simulink model "BMS_SOC_Estimation"  (R2026a)
settings: Solver=FixedStepDiscrete  StopTime=SIM_STOP_TIME  FixedStep=SIM_TIMESTEP
undefined symbols (not defined in the file): C1, DiscIntNeverNeededParam, OCV_values, Q_RATED, R0, R1, SIM_TIMESTEP, SOC_breakpoints, SOC_INIT
settings Model: VariantFading=off

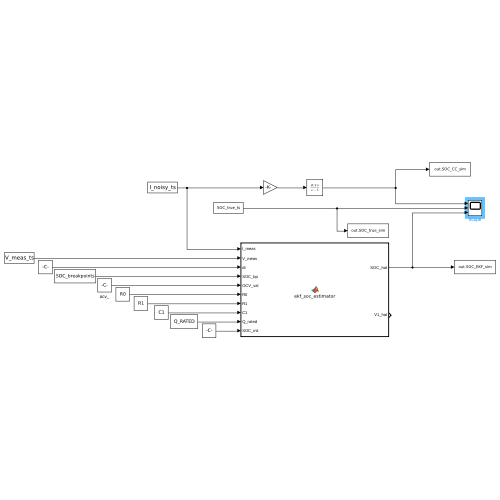
[thumbnail: Simulink's stored preview of the top-level diagram]
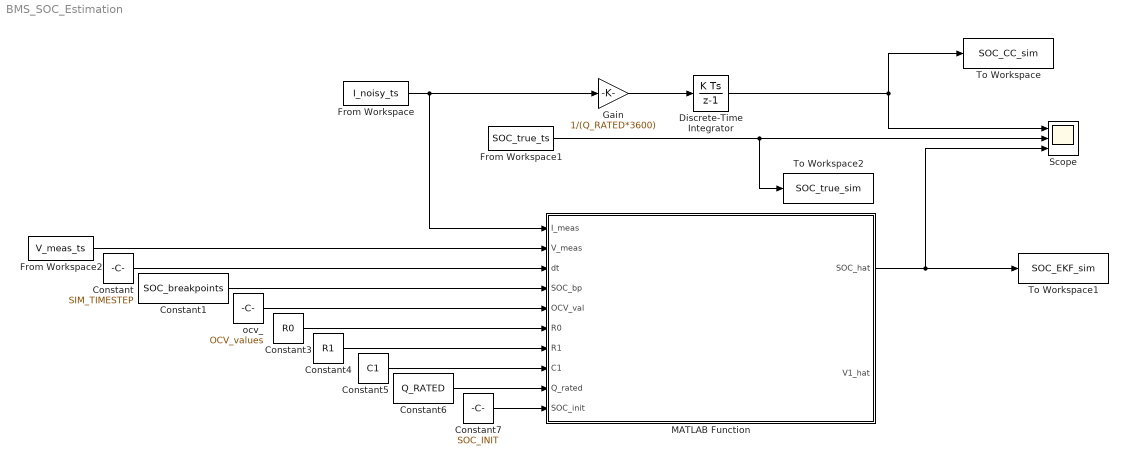
== system BMS_SOC_Estimation ==
  Constant : Constant  Value=SIM_TIMESTEP
  Constant1 : Constant  Value=SOC_breakpoints
  Constant3 : Constant  Value=R0
  Constant4 : Constant  Value=R1
  Constant5 : Constant  Value=C1
  Constant6 : Constant  Value=Q_RATED
  Constant7 : Constant  Value=SOC_INIT
  Discrete-Time Integrator : DiscreteIntegrator  InitialCondition=SOC_INIT  SampleTime=SIM_TIMESTEP  ICPrevOutput=DiscIntNeverNeededParam  ICPrevScaledInput=DiscIntNeverNeededParam
  From Workspace : FromWorkspace  VariableName=I_noisy_ts  SampleTime=SIM_TIMESTEP
  From Workspace1 : FromWorkspace  VariableName=SOC_true_ts  SampleTime=SIM_TIMESTEP
  From Workspace2 : FromWorkspace  VariableName=V_meas_ts  SampleTime=SIM_TIMESTEP
  Gain : Gain  Gain=1/(Q_RATED*3600)
  MATLAB Function : MATLAB Function  TreatAsAtomicUnit=on  SystemSampleTime=SIM_TIMESTEP
  Scope : Scope  NumInputPorts=3
      settings: ActiveDisplayYMinimum=-0.37043853989155529  ActiveDisplayYMaximum=1.9584342127717893
  To Workspace : ToWorkspace  VariableName=SOC_CC_sim  SampleTime=SIM_TIMESTEP
  To Workspace1 : ToWorkspace  VariableName=SOC_EKF_sim  SampleTime=SIM_TIMESTEP
  To Workspace2 : ToWorkspace  VariableName=SOC_true_sim  SampleTime=SIM_TIMESTEP
  ocv_ : Constant  Value=OCV_values
  wires:
  From Workspace/1 -> MATLAB Function/1(I_meas), Gain/1
  From Workspace1/1 -> Scope/2, To Workspace2/1
  From Workspace2/1 -> MATLAB Function/2(V_meas)
  Constant/1 -> MATLAB Function/3(dt)
  Constant1/1 -> MATLAB Function/4(SOC_bp)
  ocv_/1 -> MATLAB Function/5(OCV_val)
  Constant3/1 -> MATLAB Function/6(R0)
  Constant4/1 -> MATLAB Function/7(R1)
  Constant5/1 -> MATLAB Function/8(C1)
  Constant6/1 -> MATLAB Function/9(Q_rated)
  Constant7/1 -> MATLAB Function/10(SOC_init)
  Gain/1 -> Discrete-Time Integrator/1
  Discrete-Time Integrator/1 -> Scope/1, To Workspace/1
  MATLAB Function/1(SOC_hat) -> Scope/3, To Workspace1/1

== matlab function BMS_SOC_Estimation/MATLAB Function ==
  data: I_meas input; SOC_hat output; V_meas input; dt input; SOC_bp input; OCV_val input; R0 input; R1 input; C1 input; Q_rated input; SOC_init input; V1_hat output
function [SOC_hat, V1_hat] = ekf_soc_estimator(I_meas, V_meas, dt, SOC_bp, OCV_val, R0, R1, C1, Q_rated, SOC_init)
% EKF_SOC_ESTIMATOR  Extended Kalman Filter SOC estimator for a 1RC
% Thevenin equivalent circuit battery model.
%
% Paste this ENTIRE function body into a Simulink "MATLAB Function" block
% (Simulink Library Browser -> User-Defined Functions -> MATLAB Function).
%
% Inputs:
%   I_meas   - noisy measured current (A). Convention: negative = discharge
%   V_meas   - measured terminal voltage (V)
%   dt       - sample time (s)
%   SOC_bp   - OCV-SOC table breakpoints (vector, 0 to 1)
%   OCV_val  - OCV-SOC table values (vector, V)
%   R0       - ohmic resistance (Ohm)
%   R1       - polarization resistance (Ohm)
%   C1       - polarization capacitance (F)
%   Q_rated  - rated capacity (Ah)
%   SOC_init - initial SOC (0 to 1), used only on the first call
%
% Outputs:
%   SOC_hat  - EKF state-of-charge estimate (0 to 1)
%   V1_hat   - EKF estimate of the RC branch voltage (V)

persistent x P initialized
if isempty(initialized)
    x = [SOC_init; 0];          % state: [SOC; V1]
    P = diag([1e-4, 1e-4]);     % initial state covariance
    initialized = true;
end

tau = R1 * C1;
a = exp(-dt / tau);

% Dataset convention: I_meas is negative during discharge.
% Idis = positive during discharge (standard Thevenin-model convention).
Idis = -I_meas;

%% --- Predict step ---
SOC_pred = x(1) - (dt / (Q_rated * 3600)) * Idis;
V1_pred  = a * x(2) + R1 * (1 - a) * Idis;
x_pred = [SOC_pred; V1_pred];

F = [1, 0; 0, a];               % Jacobian of process model wrt state
Qcov = diag([1e-9, 1e-5]);      % process noise covariance (tuned via grid search,
% cross-validated across UDDS + US06 for robustness)
P_pred = F * P * F' + Qcov;

%% --- Measurement update step ---
OCV_pred = interp1(SOC_bp, OCV_val, x_pred(1), 'linear', 'extrap');

% Numerical gradient of OCV wrt SOC, for the measurement Jacobian
dSOC = 1e-4;
OCV_p = interp1(SOC_bp, OCV_val, x_pred(1) + dSOC, 'linear', 'extrap');
OCV_m = interp1(SOC_bp, OCV_val, x_pred(1) - dSOC, 'linear', 'extrap');
dOCV_dSOC = (OCV_p - OCV_m) / (2 * dSOC);

H = [dOCV_dSOC, -1];            % Jacobian of measurement model wrt state
Vt_pred = OCV_pred - Idis * R0 - x_pred(2);

Rcov = 8.0;                     % measurement noise variance (tuned; deliberately
% high -- see project notes: low Rcov overfit to
% gentle drive cycles and overcorrected on
% aggressive ones like US06)
y = V_meas - Vt_pred;           % innovation (measurement residual)
S = H * P_pred * H' + Rcov;
K = P_pred * H' / S;            % Kalman gain

x_upd = x_pred + K * y;
P_upd = (eye(2) - K * H) * P_pred;

% Keep SOC physically valid
x_upd(1) = min(max(x_upd(1), 0), 1);

x = x_upd;
P = P_upd;

SOC_hat = x(1);
V1_hat  = x(2);
end
